simulink model "torqueControlBalancing"  (Simulink 9.1)
settings: Solver=FixedStepDiscrete  StartTime=0.0  StopTime="Config.SIMULATION_TIME "  FixedStep=Config.tStep  RelTol=1e-3  EnableMultiTasking=on
PostLoadFcn:
  | %% Try to open the static GUI and try to adjust it
  | try
  | 
  |     staticGUI = simulinkStaticGUI;
  | 
  | end
InitFcn:
  | %% initialize the simulation
  | cd(fileparts(which(bdroot)));
  | initTorqueControlBalancing;
  | 
  | %% Try to edit the GUI (the user may have already closed it)
  | try
  | 
  |     %% Update Start Button
  |     set(sl_synch_handles.startButton,'Backgroundcolor',[0.0,1.0,0.0]);
  |     set(sl_synch_handles.startButton,'Enable','on');
  | 
  | end
StartFcn:
  | %% Try to edit the GUI (the user may have already closed it)
  | try
  | 
  |     %% Update Start Button
  |     set(sl_synch_handles.startButton,'Backgroundcolor',[0.8,0.8,0.8]);
  |     set(sl_synch_handles.startButton,'Enable','off');
  | 
  |     %% Update Compile Button
  |     set(sl_synch_handles.compileButton,'Backgroundcolor',[0.8,0.8,0.8]);
  |     set(sl_synch_handles.compileButton,'Enable','off');
  | 
  |     %% Update Exit Button
  |     set(sl_synch_handles.exitButton,'Backgroundcolor',[0.8,0.8,0.8]);
  |     set(sl_synch_handles.exitButton,'Enable','off');
  | 
  | end
StopFcn:
  | %% stop the simulation
  | cd(fileparts(which(bdroot)));
  | stopTorqueControlBalancing;
  | 
  | %% Try to edit the GUI (the user may have already closed it)
  | try
  | 
  |     %% Update Compile Button
  |     set(sl_synch_handles.compileButton,'Backgroundcolor',[1.0,0.6,0.0]);
  |     set(sl_synch_handles.compileButton,'Enable','on');
  | 
  |     %% Update Exit Button
  |     set(sl_synch_handles.exitButton,'Backgroundcolor',[0.0,1.0,1.0]);
  |     set(sl_synch_handles.exitButton,'Enable','on');
  | 
  | end
undefined symbols (not defined in the file or in its folder): bVectorConstraints, Config, ConstraintsMatrix, Gain, Reg, ROBOT_DOF, Sat, StateMachine
libraries: WBToolboxLibrary x77
(part 2 of 2)

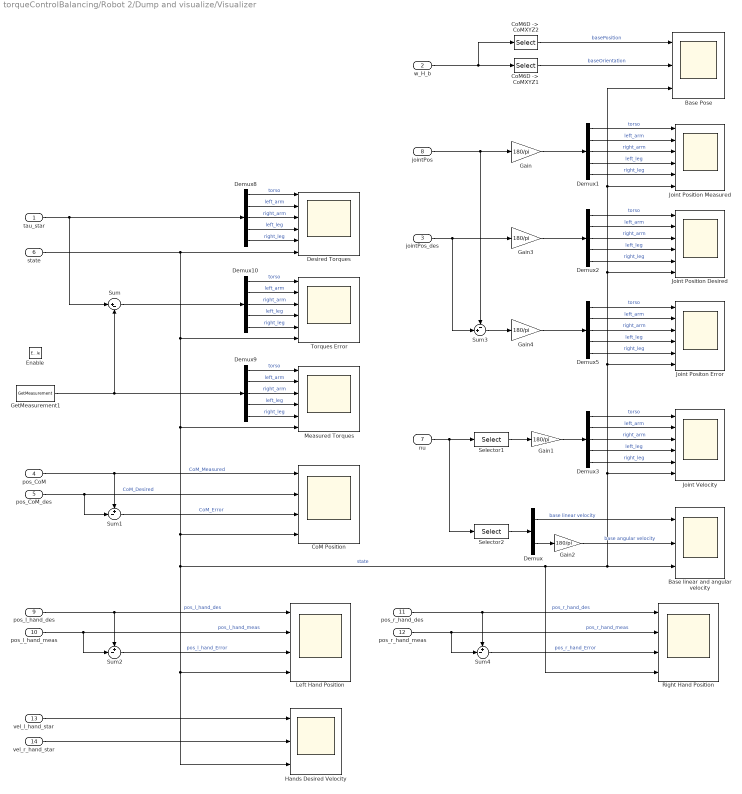
== system torqueControlBalancing/Robot 2/Dump and visualize/Visualizer ==
  tau_star : Inport
  w_H_b : Inport  Port=2
  jointPos_des : Inport  Port=3
  pos_CoM : Inport  Port=4
  pos_CoM_des : Inport  Port=5
  state : Inport  Port=6
  nu : Inport  Port=7
  jointPos : Inport  Port=8
  pos_l_hand_des : Inport  Port=9
  pos_l_hand_meas : Inport  Port=10
  pos_r_hand_des : Inport  Port=11
  pos_r_hand_meas : Inport  Port=12
  vel_l_hand_star : Inport  Port=13
  vel_r_hand_star : Inport  Port=14
  Enable : EnablePort
  Base Pose : Scope  NumInputPorts=3
  Base linear and angular velocity : Scope  NumInputPorts=3
  CoM Position : Scope  NumInputPorts=4
  "CoM6D ->  CoMXYZ1" : Selector  NumberOfDimensions=2  InputPortWidth=7  IndexOptions=Index vector (dialog),Index vector (dialog)  Indices=[1 2 3],[1 2 3]  OutputSizes=1,1
  "CoM6D ->  CoMXYZ2" : Selector  NumberOfDimensions=2  InputPortWidth=7  IndexOptions=Index vector (dialog),Index vector (dialog)  Indices=[1 2 3],[4]  OutputSizes=1,1
  Demux : Demux  Outputs=2
  Demux{1..3,5,8..10} (7 alike) : Demux  Outputs=Config.numOfJointsForEachControlboard
  Desired Torques : Scope  NumInputPorts=6
  Gain{,1..4} (5 alike) : Gain  Gain=180/pi
  GetMeasurement1 : WBToolboxLibrary/States/GetMeasurement  measuredType=Joints Torque
      settings: SourceProductName=WholeBodyToolbox
  Hands Desired Velocity : Scope  NumInputPorts=3
  Joint Position Desired : Scope  NumInputPorts=6
  Joint Position Measured : Scope  NumInputPorts=6
  Joint Positon Error : Scope  NumInputPorts=6
  Joint Velocity : Scope  NumInputPorts=6
  Left Hand Position : Scope  NumInputPorts=4
  Measured Torques : Scope  NumInputPorts=6
  Right Hand Position : Scope  NumInputPorts=4
  Selector1 : Selector  InputPortWidth=6+ROBOT_DOF  IndexOptions=Index vector (dialog)  Indices=[7:6+ROBOT_DOF]  OutputSizes=1
  Selector2 : Selector  InputPortWidth=6+ROBOT_DOF  IndexOptions=Index vector (dialog)  Indices=[1:6]  OutputSizes=1
  Sum : Sum  Inputs=|+-
  Sum1 : Sum  Inputs=+-|
  Sum2 : Sum  Inputs=+-|
  Sum3 : Sum  Inputs=-+|
  Sum4 : Sum  Inputs=+-|
  Torques Error : Scope  NumInputPorts=6
  wires:
  pos_CoM/1 -> Sum1/1, CoM Position/1  "CoM_Measured"
  Gain/1 -> Demux1/1
  jointPos/1 -> Gain/1, Sum3/1
  Demux1/5 -> Joint Position Measured/5  "right_leg"
  Demux1/1 -> Joint Position Measured/1  "torso"
  Demux1/2 -> Joint Position Measured/2  "left_arm"
  Demux1/4 -> Joint Position Measured/4  "left_leg"
  Demux1/3 -> Joint Position Measured/3  "right_arm"
  GetMeasurement1/1 -> Sum/2, Demux9/1
  Demux8/5 -> Desired Torques/5  "right_leg"
  Demux8/1 -> Desired Torques/1  "torso"
  Demux8/2 -> Desired Torques/2  "left_arm"
  Demux8/4 -> Desired Torques/4  "left_leg"
  Demux8/3 -> Desired Torques/3  "right_arm"
  Demux10/5 -> Torques Error/5  "right_leg"
  Demux10/1 -> Torques Error/1  "torso"
  Demux10/2 -> Torques Error/2  "left_arm"
  Demux10/4 -> Torques Error/4  "left_leg"
  Demux10/3 -> Torques Error/3  "right_arm"
  Sum/1 -> Demux10/1
  Demux9/5 -> Measured Torques/5  "right_leg"
  Demux9/1 -> Measured Torques/1  "torso"
  Demux9/2 -> Measured Torques/2  "left_arm"
  Demux9/4 -> Measured Torques/4  "left_leg"
  Demux9/3 -> Measured Torques/3  "right_arm"
  jointPos_des/1 -> Sum3/2, Gain3/1
  Gain3/1 -> Demux2/1
  Demux2/5 -> Joint Position Desired/5  "right_leg"
  Demux2/1 -> Joint Position Desired/1  "torso"
  Demux2/2 -> Joint Position Desired/2  "left_arm"
  Demux2/4 -> Joint Position Desired/4  "left_leg"
  Demux2/3 -> Joint Position Desired/3  "right_arm"
  Gain4/1 -> Demux5/1
  Demux5/5 -> Joint Positon Error/5  "right_leg"
  Demux5/1 -> Joint Positon Error/1  "torso"
  Demux5/2 -> Joint Positon Error/2  "left_arm"
  Demux5/4 -> Joint Positon Error/4  "left_leg"
  Demux5/3 -> Joint Positon Error/3  "right_arm"
  Sum3/1 -> Gain4/1
  pos_CoM_des/1 -> Sum1/2, CoM Position/2  "CoM_Desired"
  w_H_b/1 -> "CoM6D ->  CoMXYZ2"/1, "CoM6D ->  CoMXYZ1"/1
  "CoM6D ->  CoMXYZ2"/1 -> Base Pose/1  "basePosition"
  "CoM6D ->  CoMXYZ1"/1 -> Base Pose/2  "baseOrientation"
  tau_star/1 -> Sum/1, Demux8/1
  nu/1 -> Selector1/1, Selector2/1
  Selector2/1 -> Demux/1
  Gain1/1 -> Demux3/1
  Demux/1 -> Base linear and angular velocity/1  "base linear velocity"
  Gain2/1 -> Base linear and angular velocity/2  "base angular velocity"
  Demux3/3 -> Joint Velocity/3  "right_arm"
  Demux3/5 -> Joint Velocity/5  "right_leg"
  Selector1/1 -> Gain1/1
  Demux3/1 -> Joint Velocity/1  "torso"
  Demux3/2 -> Joint Velocity/2  "left_arm"
  Demux3/4 -> Joint Velocity/4  "left_leg"
  Demux/2 -> Gain2/1
  Sum1/1 -> CoM Position/3  "CoM_Error"
  pos_l_hand_des/1 -> Left Hand Position/1, Sum2/1  "pos_l_hand_des"
  pos_l_hand_meas/1 -> Sum2/2, Left Hand Position/2  "pos_l_hand_meas"
  Sum2/1 -> Left Hand Position/3  "pos_l_hand_Error"
  pos_r_hand_meas/1 -> Sum4/2, Right Hand Position/2  "pos_r_hand_meas"
  pos_r_hand_des/1 -> Right Hand Position/1, Sum4/1  "pos_r_hand_des"
  state/1 -> Left Hand Position/4, Hands Desired Velocity/3, Right Hand Position/4, Base linear and angular velocity/3, Joint Velocity/6, Joint Positon Error/6, Joint Position Desired/6, Base Pose/3, Joint Position Measured/6, CoM Position/4, Measured Torques/6, Torques Error/6, Desired Torques/6  "state"
  Sum4/1 -> Right Hand Position/3  "pos_r_hand_Error"
  vel_l_hand_star/1 -> Hands Desired Velocity/1
  vel_r_hand_star/1 -> Hands Desired Velocity/2

== system torqueControlBalancing/Robot 2/Dynamics and Kinematics/Dynamics ==
  w_H_b : Inport
  jointPos : Inport  Port=2
  nu : Inport  Port=3
  CentroidalMomentum : WBToolboxLibrary/Model/Dynamics/CentroidalMomentum
      settings: SourceProductName=WholeBodyToolbox
  "CoM6D ->  CoMXYZ1" : Selector  InputPortWidth=6+ROBOT_DOF  IndexOptions=Index vector (dialog)  Indices=[7:6+ROBOT_DOF]  OutputSizes=1
  "CoM6D ->  CoMXYZ2" : Selector  InputPortWidth=6+ROBOT_DOF  IndexOptions=Index vector (dialog)  Indices=[1 2 3 4 5 6]  OutputSizes=1
  GetBiasForces : WBToolboxLibrary/Model/Dynamics/GetBiasForces
      settings: SourceProductName=WholeBodyToolbox
  MassMatrix : WBToolboxLibrary/Model/Dynamics/MassMatrix
      settings: SourceProductName=WholeBodyToolbox
  M : Outport
  h : Outport  Port=2
  L : Outport  Port=3
  wires:
  CentroidalMomentum/1 -> L/1
  GetBiasForces/1 -> h/1
  w_H_b/1 -> CentroidalMomentum/1, GetBiasForces/1, MassMatrix/1
  jointPos/1 -> CentroidalMomentum/2, GetBiasForces/2, MassMatrix/2
  "CoM6D ->  CoMXYZ2"/1 -> CentroidalMomentum/3, GetBiasForces/3
  "CoM6D ->  CoMXYZ1"/1 -> CentroidalMomentum/4, GetBiasForces/4
  nu/1 -> "CoM6D ->  CoMXYZ1"/1, "CoM6D ->  CoMXYZ2"/1
  MassMatrix/1 -> M/1

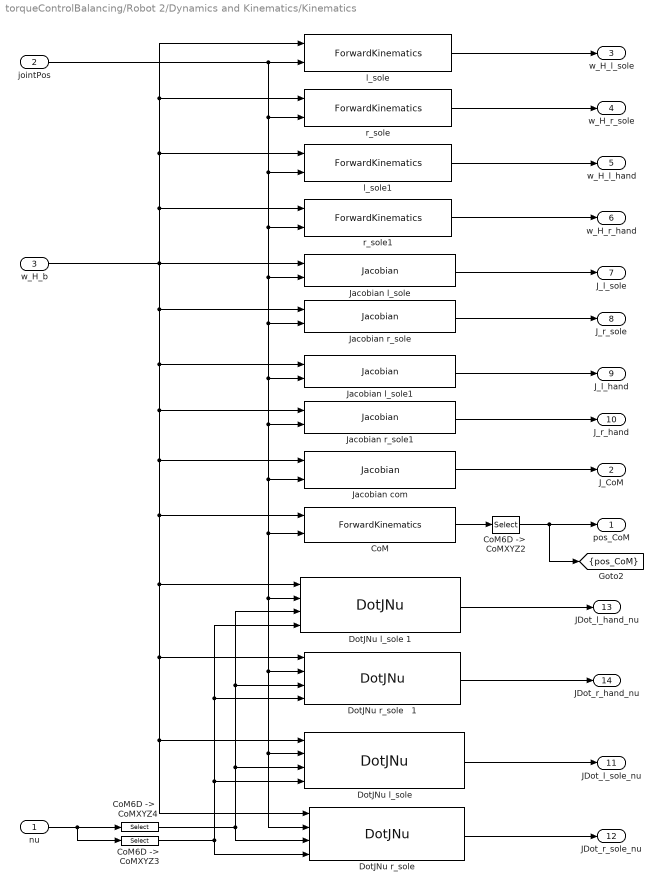
== system torqueControlBalancing/Robot 2/Dynamics and Kinematics/Kinematics ==
  nu : Inport
  jointPos : Inport  Port=2
  w_H_b : Inport  Port=3
  CoM : WBToolboxLibrary/Model/Kinematics/ForwardKinematics  frameName=Frames.COM
      settings: SourceProductName=WholeBodyToolbox
  "CoM6D ->  CoMXYZ2" : Selector  NumberOfDimensions=2  InputPortWidth=7  IndexOptions=Index vector (dialog),Index vector (dialog)  Indices=[1 2 3],[4]  OutputSizes=1,1
  "CoM6D ->  CoMXYZ3" : Selector  InputPortWidth=6+ROBOT_DOF  IndexOptions=Index vector (dialog)  Indices=[7:6+ROBOT_DOF]  OutputSizes=1
  "CoM6D ->  CoMXYZ4" : Selector  InputPortWidth=6+ROBOT_DOF  IndexOptions=Index vector (dialog)  Indices=[1 2 3 4 5 6]  OutputSizes=1
  "DotJNu l_sole " : WBToolboxLibrary/Model/Jacobians/DotJNu  frameName=Frames.LEFT_FOOT
      settings: SourceProductName=WholeBodyToolbox
  DotJNu l_sole 1 : WBToolboxLibrary/Model/Jacobians/DotJNu  frameName=Frames.LEFT_HAND
      settings: SourceProductName=WholeBodyToolbox
  "DotJNu r_sole   " : WBToolboxLibrary/Model/Jacobians/DotJNu  frameName=Frames.RIGHT_FOOT
      settings: SourceProductName=WholeBodyToolbox
  DotJNu r_sole   1 : WBToolboxLibrary/Model/Jacobians/DotJNu  frameName=Frames.RIGHT_HAND
      settings: SourceProductName=WholeBodyToolbox
  Jacobian com : WBToolboxLibrary/Model/Jacobians/Jacobian  frameName=Frames.COM
      settings: SourceProductName=WholeBodyToolbox
  Jacobian l_sole : WBToolboxLibrary/Model/Jacobians/Jacobian  frameName=Frames.LEFT_FOOT
      settings: SourceProductName=WholeBodyToolbox
  Jacobian l_sole1 : WBToolboxLibrary/Model/Jacobians/Jacobian  frameName=Frames.LEFT_HAND
      settings: SourceProductName=WholeBodyToolbox
  Jacobian r_sole : WBToolboxLibrary/Model/Jacobians/Jacobian  frameName=Frames.RIGHT_FOOT
      settings: SourceProductName=WholeBodyToolbox
  Jacobian r_sole1 : WBToolboxLibrary/Model/Jacobians/Jacobian  frameName=Frames.RIGHT_HAND
      settings: SourceProductName=WholeBodyToolbox
  l_sole : WBToolboxLibrary/Model/Kinematics/ForwardKinematics  frameName=Frames.LEFT_FOOT
      settings: SourceProductName=WholeBodyToolbox
  l_sole1 : WBToolboxLibrary/Model/Kinematics/ForwardKinematics  frameName=Frames.LEFT_HAND
      settings: SourceProductName=WholeBodyToolbox
  r_sole : WBToolboxLibrary/Model/Kinematics/ForwardKinematics  frameName=Frames.RIGHT_FOOT
      settings: SourceProductName=WholeBodyToolbox
  r_sole1 : WBToolboxLibrary/Model/Kinematics/ForwardKinematics  frameName=Frames.RIGHT_HAND
      settings: SourceProductName=WholeBodyToolbox
  pos_CoM : Outport
  J_CoM : Outport  Port=2
  w_H_l_sole : Outport  Port=3
  w_H_r_sole : Outport  Port=4
  w_H_l_hand : Outport  Port=5
  w_H_r_hand : Outport  Port=6
  J_l_sole : Outport  Port=7
  J_r_sole : Outport  Port=8
  J_l_hand : Outport  Port=9
  J_r_hand : Outport  Port=10
  JDot_l_sole_nu : Outport  Port=11
  JDot_r_sole_nu : Outport  Port=12
  JDot_l_hand_nu : Outport  Port=13
  JDot_r_hand_nu : Outport  Port=14
  tag scope: pos_CoM=scoped
  wires:
  "CoM6D ->  CoMXYZ3"/1 -> "DotJNu r_sole   "/4, DotJNu l_sole 1/4, DotJNu r_sole   1/4, "DotJNu l_sole "/4
  "CoM6D ->  CoMXYZ4"/1 -> "DotJNu r_sole   "/3, DotJNu r_sole   1/3, DotJNu l_sole 1/3, "DotJNu l_sole "/3
  nu/1 -> "CoM6D ->  CoMXYZ3"/1, "CoM6D ->  CoMXYZ4"/1
  l_sole/1 -> w_H_l_sole/1
  r_sole/1 -> w_H_r_sole/1
  Jacobian l_sole/1 -> J_l_sole/1
  Jacobian r_sole/1 -> J_r_sole/1
  Jacobian com/1 -> J_CoM/1
  CoM/1 -> "CoM6D ->  CoMXYZ2"/1
  "DotJNu l_sole "/1 -> JDot_l_sole_nu/1
  "DotJNu r_sole   "/1 -> JDot_r_sole_nu/1
  "CoM6D ->  CoMXYZ2"/1 -> [pos_CoM], pos_CoM/1
  Jacobian l_sole1/1 -> J_l_hand/1
  Jacobian r_sole1/1 -> J_r_hand/1
  w_H_b/1 -> Jacobian l_sole1/1, Jacobian com/1, DotJNu l_sole 1/1, DotJNu r_sole   1/1, "DotJNu r_sole   "/1, "DotJNu l_sole "/1, CoM/1, Jacobian r_sole1/1, Jacobian r_sole/1, Jacobian l_sole/1, r_sole1/1, l_sole1/1, r_sole/1, l_sole/1
  r_sole1/1 -> w_H_r_hand/1
  l_sole1/1 -> w_H_l_hand/1
  jointPos/1 -> l_sole1/2, r_sole1/2, Jacobian l_sole1/2, Jacobian r_sole1/2, Jacobian com/2, DotJNu l_sole 1/2, DotJNu r_sole   1/2, "DotJNu r_sole   "/2, "DotJNu l_sole "/2, CoM/2, Jacobian r_sole/2, Jacobian l_sole/2, r_sole/2, l_sole/2
  DotJNu r_sole   1/1 -> JDot_r_hand_nu/1
  DotJNu l_sole 1/1 -> JDot_l_hand_nu/1

== system torqueControlBalancing/Robot 2/Robot State and References/Compute State Velocity ==
  jointPos : Inport
  jointVel : Inport  Port=2
  w_H_b : Inport  Port=3
  Compute Base Velocity : MATLAB Function  TreatAsAtomicUnit=on
  Feet Jacobians : Subsystem
  Mux : Mux  Inputs=2
  nu : Outport
  wires:
  jointVel/1 -> Mux/2, Compute Base Velocity/3(jointVel)
  Mux/1 -> nu/1
  Compute Base Velocity/1(nu_b) -> Mux/1
  jointPos/1 -> Feet Jacobians/1(jointPos)
  w_H_b/1 -> Feet Jacobians/2(w_H_b)
  Feet Jacobians/1(J_l_sole) -> Compute Base Velocity/1(J_l_sole)
  Feet Jacobians/2(J_r_sole) -> Compute Base Velocity/2(J_r_sole)

== system torqueControlBalancing/Robot 2/Robot State and References/Compute base to fixed link transform ==
  jointPos : Inport
  Constant7 : Constant  Value=eye(4)
  "LFoot to base link transform " : Subsystem
  Relative transform l_sole_H_base : WBToolboxLibrary/Model/Kinematics/ForwardKinematics  frameName=Frames.LEFT_FOOT
      settings: SourceProductName=WholeBodyToolbox
  fixed_l_sole_H_b : Outport
  tag scope: jointPos=scoped
  wires:
  Constant7/1 -> "LFoot to base link transform "/3(w_H_base_fixed), Relative transform l_sole_H_base/1
  "LFoot to base link transform "/1(link_H_b) -> fixed_l_sole_H_b/1
  Relative transform l_sole_H_base/1 -> "LFoot to base link transform "/2(w_H_link)
  jointPos/1 -> [jointPos], "LFoot to base link transform "/1(jointPos), Relative transform l_sole_H_base/2

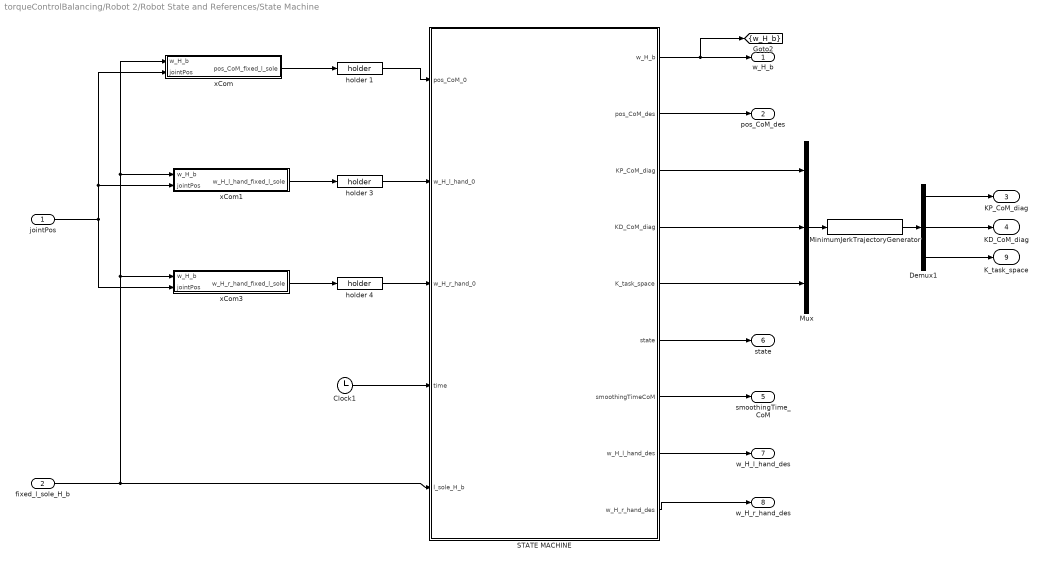
== system torqueControlBalancing/Robot 2/Robot State and References/State Machine ==
  jointPos : Inport
  fixed_l_sole_H_b : Inport  Port=2
  Clock1 : Clock
  Demux1 : Demux  Outputs=[3,3,2]
  MinimumJerkTrajectoryGenerator : WBToolboxLibrary/Utilities/MinimumJerkTrajectoryGenerator  externalSettlingTime=off  settlingTime=Config.SmoothingTimeGainScheduling  sampleTime=Config.tStep  resetOnSettlingTime=off  firstDerivatives=off  secondDerivatives=off  explicitInitialValue=off
      settings: SourceProductName=WholeBodyToolbox
  Mux : Mux  Inputs=3
  STATE MACHINE : MATLAB Function  TreatAsAtomicUnit=on
  holder 1 : WBToolboxLibrary/Utilities/holder 
      settings: SourceProductName=WholeBodyToolbox
  holder 3 : WBToolboxLibrary/Utilities/holder 
      settings: SourceProductName=WholeBodyToolbox
  holder 4 : WBToolboxLibrary/Utilities/holder 
      settings: SourceProductName=WholeBodyToolbox
  xCom : Subsystem
  xCom1 : Subsystem
  xCom3 : Subsystem
  w_H_b : Outport
  pos_CoM_des : Outport  Port=2
  KP_CoM_diag : Outport  Port=3
  KD_CoM_diag : Outport  Port=4
  smoothingTime_CoM : Outport  Port=5
  state : Outport  Port=6
  w_H_l_hand_des : Outport  Port=7
  w_H_r_hand_des : Outport  Port=8
  K_task_space : Outport  Port=9
  tag scope: w_H_b=scoped
  wires:
  xCom/1("pos_CoM_fixed_l_sole ") -> holder 1/1
  STATE MACHINE/2(pos_CoM_des) -> pos_CoM_des/1
  STATE MACHINE/6(state) -> state/1
  STATE MACHINE/3(KP_CoM_diag) -> Mux/1
  STATE MACHINE/4(KD_CoM_diag) -> Mux/2
  Mux/1 -> MinimumJerkTrajectoryGenerator/1
  MinimumJerkTrajectoryGenerator/1 -> Demux1/1
  jointPos/1 -> xCom1/2(jointPos), xCom/2(jointPos), xCom3/2(jointPos)
  fixed_l_sole_H_b/1 -> xCom/1(w_H_b), xCom1/1(w_H_b), xCom3/1(w_H_b), STATE MACHINE/5(l_sole_H_b)
  Clock1/1 -> STATE MACHINE/4(time)
  holder 1/1 -> STATE MACHINE/1(pos_CoM_0)
  STATE MACHINE/7(smoothingTimeCoM) -> smoothingTime_CoM/1
  STATE MACHINE/1(w_H_b) -> [w_H_b], w_H_b/1
  xCom1/1("w_H_l_hand_fixed_l_sole ") -> holder 3/1
  holder 3/1 -> STATE MACHINE/2(w_H_l_hand_0)
  xCom3/1("w_H_r_hand_fixed_l_sole ") -> holder 4/1
  holder 4/1 -> STATE MACHINE/3(w_H_r_hand_0)
  STATE MACHINE/5(K_task_space) -> Mux/3
  STATE MACHINE/8(w_H_l_hand_des) -> w_H_l_hand_des/1
  STATE MACHINE/9(w_H_r_hand_des) -> w_H_r_hand_des/1
  Demux1/1 -> KP_CoM_diag/1
  Demux1/2 -> KD_CoM_diag/1
  Demux1/3 -> K_task_space/1

== system torqueControlBalancing/Robot 2/Robot State and References/Update Gains and References ==
  pos_CoM_des : Inport
  KP_CoM_diag : Inport  Port=2
  KD_CoM_diag : Inport  Port=3
  smoothingTime_CoM : Inport  Port=4
  Reshape Gains Matrices : Subsystem
  Selector1 : Selector  NumberOfDimensions=2  InputPortWidth=3  IndexOptions=Index vector (dialog),Index vector (dialog)  Indices=[1 2 3],[1]  OutputSizes=1,1
  Smooth reference CoM : Subsystem
  KP_CoM : Outport
  KD_CoM : Outport  Port=2
  desired_pos_vel_acc_CoM : Outport  Port=3
  tag scope: pos_CoM_des=scoped
  wires:
  pos_CoM_des/1 -> Smooth reference CoM/1(pos_CoM_des)
  smoothingTime_CoM/1 -> Smooth reference CoM/2(smoothingTime_CoM)
  Smooth reference CoM/1(desired_pos_vel_acc_CoM) -> Selector1/1, desired_pos_vel_acc_CoM/1
  KP_CoM_diag/1 -> Reshape Gains Matrices/1(KP_CoM_diag)
  KD_CoM_diag/1 -> Reshape Gains Matrices/2(KD_CoM_diag)
  Reshape Gains Matrices/1(KP_CoM) -> KP_CoM/1
  Reshape Gains Matrices/2(KD_CoM) -> KD_CoM/1
  Selector1/1 -> [pos_CoM_des]

== system torqueControlBalancing/Robot 2/emergency stop: joint limits/STOP IF JOINTS HIT THE LIMITS ==
  jointPos : Inport
  Enable : EnablePort
  Assertion : Assertion
  GetLimits : WBToolboxLibrary/States/GetLimits  limitsSource=ControlBoard  limitsType=Position
      settings: SourceProductName=WholeBodyToolbox
  MATLAB Function : MATLAB Function  TreatAsAtomicUnit=on
  index1 : Constant  Value=0.01  VectorParams1D=off
  wires:
  jointPos/1 -> MATLAB Function/3(u)
  MATLAB Function/1(inRange) -> Assertion/1
  GetLimits/1 -> MATLAB Function/1(umin)
  GetLimits/2 -> MATLAB Function/2(umax)
  index1/1 -> MATLAB Function/4(tol)

== system torqueControlBalancing/Robot 2/emergency stop: joint limits/STOP IF THERE ARE SPIKES IN THE ENCODERS ==
  jointPos : Inport
  Enable : EnablePort
  Assertion : Assertion
  MATLAB Function : MATLAB Function  TreatAsAtomicUnit=on
  index1 : Constant  Value=Sat.maxJointsPositionDelta  VectorParams1D=off
  wires:
  jointPos/1 -> MATLAB Function/1(u)
  MATLAB Function/1(noSpikes) -> Assertion/1
  index1/1 -> MATLAB Function/2(delta_u_max)

== system torqueControlBalancing/Robot 1/Balancing Controller QP/Compute Desired Torques/QPSolver ==
  HessianMatrixTwoFeet : Inport
  gradientTwoFeet : Inport  Port=2
  ConstraintsMatrixTwoFeet : Inport  Port=3
  bVectorConstraintsTwoFeet : Inport  Port=4
  QP Two Feet : Subsystem  TreatAsAtomicUnit=on
  f_0_twoFeet : Outport
  tag scope: QPStatus=scoped
  wires:
  bVectorConstraintsTwoFeet/1 -> QP Two Feet/4(ubA)
  gradientTwoFeet/1 -> QP Two Feet/2(g)
  ConstraintsMatrixTwoFeet/1 -> QP Two Feet/3(A)
  HessianMatrixTwoFeet/1 -> QP Two Feet/1(H)
  QP Two Feet/1(QPStatus) -> [QPStatus]
  QP Two Feet/2(f0_twoFeet) -> f_0_twoFeet/1

== system torqueControlBalancing/Robot 1/Robot State and References/Compute State Velocity/Feet Jacobians ==
  jointPos : Inport
  w_H_b : Inport  Port=2
  Jacobian l_sole : WBToolboxLibrary/Model/Jacobians/Jacobian  frameName=Frames.LEFT_FOOT
      settings: SourceProductName=WholeBodyToolbox
  Jacobian r_sole : WBToolboxLibrary/Model/Jacobians/Jacobian  frameName=Frames.RIGHT_FOOT
      settings: SourceProductName=WholeBodyToolbox
  J_l_sole : Outport
  J_r_sole : Outport  Port=2
  wires:
  Jacobian l_sole/1 -> J_l_sole/1
  Jacobian r_sole/1 -> J_r_sole/1
  w_H_b/1 -> Jacobian r_sole/1, Jacobian l_sole/1
  jointPos/1 -> Jacobian l_sole/2, Jacobian r_sole/2

== system torqueControlBalancing/Robot 1/Robot State and References/Compute base to fixed link transform/LFoot to base link transform  ==
  jointPos : Inport
  w_H_link : Inport  Port=2
  w_H_base_fixed : Inport  Port=3
  Fixed base to root link transform : WBToolboxLibrary/Model/Kinematics/ForwardKinematics  frameName=Frames.BASE
      settings: SourceProductName=WholeBodyToolbox
  Inv_2 : Product  Inputs=/*  Multiplication=Matrix(*)
  link_H_b : Outport
  wires:
  jointPos/1 -> Fixed base to root link transform/2
  Fixed base to root link transform/1 -> Inv_2/2
  w_H_link/1 -> Inv_2/1
  w_H_base_fixed/1 -> Fixed base to root link transform/1
  Inv_2/1 -> link_H_b/1  "link_H_root"

== system torqueControlBalancing/Robot 1/Robot State and References/State Machine/xCom ==
  w_H_b : Inport
  jointPos : Inport  Port=2
  CoM : WBToolboxLibrary/Model/Kinematics/ForwardKinematics  frameName=Frames.COM
      settings: SourceProductName=WholeBodyToolbox
  "CoM6D ->  CoMXYZ2" : Selector  NumberOfDimensions=2  InputPortWidth=7  IndexOptions=Index vector (dialog),Index vector (dialog)  Indices=[1 2 3],[4]  OutputSizes=1,1
  "pos_CoM_fixed_l_sole " : Outport
  wires:
  jointPos/1 -> CoM/2
  "CoM6D ->  CoMXYZ2"/1 -> "pos_CoM_fixed_l_sole "/1
  CoM/1 -> "CoM6D ->  CoMXYZ2"/1
  w_H_b/1 -> CoM/1

== system torqueControlBalancing/Robot 1/Robot State and References/State Machine/xCom1 ==
  w_H_b : Inport
  jointPos : Inport  Port=2
  Left Hand : WBToolboxLibrary/Model/Kinematics/ForwardKinematics  frameName=Frames.LEFT_HAND
      settings: SourceProductName=WholeBodyToolbox
  "w_H_l_hand_fixed_l_sole " : Outport
  wires:
  jointPos/1 -> Left Hand/2
  Left Hand/1 -> "w_H_l_hand_fixed_l_sole "/1
  w_H_b/1 -> Left Hand/1

== system torqueControlBalancing/Robot 1/Robot State and References/State Machine/xCom3 ==
  w_H_b : Inport
  jointPos : Inport  Port=2
  Right Hand : WBToolboxLibrary/Model/Kinematics/ForwardKinematics  frameName=Frames.RIGHT_HAND
      settings: SourceProductName=WholeBodyToolbox
  "w_H_r_hand_fixed_l_sole " : Outport
  wires:
  jointPos/1 -> Right Hand/2
  Right Hand/1 -> "w_H_r_hand_fixed_l_sole "/1
  w_H_b/1 -> Right Hand/1

== system torqueControlBalancing/Robot 1/Robot State and References/Update Gains and References/Reshape Gains Matrices ==
  KP_CoM_diag : Inport
  KD_CoM_diag : Inport  Port=2
  MATLAB Function1 : MATLAB Function  TreatAsAtomicUnit=on
  MATLAB Function2 : MATLAB Function  TreatAsAtomicUnit=on
  KP_CoM : Outport
  KD_CoM : Outport  Port=2
  wires:
  KP_CoM_diag/1 -> MATLAB Function1/1(d)
  KD_CoM_diag/1 -> MATLAB Function2/1(d)
  MATLAB Function1/1(D) -> KP_CoM/1
  MATLAB Function2/1(D) -> KD_CoM/1

== system torqueControlBalancing/Robot 1/Robot State and References/Update Gains and References/Smooth reference CoM ==
  pos_CoM_des : Inport
  smoothingTime_CoM : Inport  Port=2
  Constant : Constant  Value=zeros(6,1)
  MinimumJerkTrajectoryGenerator2 : WBToolboxLibrary/Utilities/MinimumJerkTrajectoryGenerator  externalSettlingTime=on  settlingTime=0.01  sampleTime=Config.tStep  resetOnSettlingTime=off  firstDerivatives=on  secondDerivatives=on  explicitInitialValue=off
      settings: SourceProductName=WholeBodyToolbox
  Mux : Mux  Inputs=3
  Mux1 : Mux  Inputs=2
  Reshape : Reshape  OutputDimensionality=Customize  OutputDimensions=[3,3]
  SMOOTH_DES_COM : Constant  Value=Config.SMOOTH_COM_DES
  Switch3 : Switch  Criteria=u2 > Threshold
  desired_pos_vel_acc_CoM : Outport
  wires:
  smoothingTime_CoM/1 -> MinimumJerkTrajectoryGenerator2/2
  Switch3/1 -> Reshape/1
  pos_CoM_des/1 -> Mux1/1, MinimumJerkTrajectoryGenerator2/1
  SMOOTH_DES_COM/1 -> Switch3/2
  MinimumJerkTrajectoryGenerator2/3 -> Mux/3
  Mux/1 -> Switch3/1
  MinimumJerkTrajectoryGenerator2/2 -> Mux/2
  Reshape/1 -> desired_pos_vel_acc_CoM/1
  MinimumJerkTrajectoryGenerator2/1 -> Mux/1
  Mux1/1 -> Switch3/3
  Constant/1 -> Mux1/2

== system torqueControlBalancing/Robot 2/Balancing Controller QP/Compute Desired Torques/QPSolver ==
  HessianMatrixTwoFeet : Inport
  gradientTwoFeet : Inport  Port=2
  ConstraintsMatrixTwoFeet : Inport  Port=3
  bVectorConstraintsTwoFeet : Inport  Port=4
  QP Two Feet : Subsystem  TreatAsAtomicUnit=on
  f_0_twoFeet : Outport
  tag scope: QPStatus=scoped
  wires:
  bVectorConstraintsTwoFeet/1 -> QP Two Feet/4(ubA)
  gradientTwoFeet/1 -> QP Two Feet/2(g)
  ConstraintsMatrixTwoFeet/1 -> QP Two Feet/3(A)
  HessianMatrixTwoFeet/1 -> QP Two Feet/1(H)
  QP Two Feet/1(QPStatus) -> [QPStatus]
  QP Two Feet/2(f0_twoFeet) -> f_0_twoFeet/1

== system torqueControlBalancing/Robot 2/Robot State and References/Compute State Velocity/Feet Jacobians ==
  jointPos : Inport
  w_H_b : Inport  Port=2
  Jacobian l_sole : WBToolboxLibrary/Model/Jacobians/Jacobian  frameName=Frames.LEFT_FOOT
      settings: SourceProductName=WholeBodyToolbox
  Jacobian r_sole : WBToolboxLibrary/Model/Jacobians/Jacobian  frameName=Frames.RIGHT_FOOT
      settings: SourceProductName=WholeBodyToolbox
  J_l_sole : Outport
  J_r_sole : Outport  Port=2
  wires:
  Jacobian l_sole/1 -> J_l_sole/1
  Jacobian r_sole/1 -> J_r_sole/1
  w_H_b/1 -> Jacobian r_sole/1, Jacobian l_sole/1
  jointPos/1 -> Jacobian l_sole/2, Jacobian r_sole/2

== system torqueControlBalancing/Robot 2/Robot State and References/Compute base to fixed link transform/LFoot to base link transform  ==
  jointPos : Inport
  w_H_link : Inport  Port=2
  w_H_base_fixed : Inport  Port=3
  Fixed base to root link transform : WBToolboxLibrary/Model/Kinematics/ForwardKinematics  frameName=Frames.BASE
      settings: SourceProductName=WholeBodyToolbox
  Inv_2 : Product  Inputs=/*  Multiplication=Matrix(*)
  link_H_b : Outport
  wires:
  jointPos/1 -> Fixed base to root link transform/2
  Fixed base to root link transform/1 -> Inv_2/2
  w_H_link/1 -> Inv_2/1
  w_H_base_fixed/1 -> Fixed base to root link transform/1
  Inv_2/1 -> link_H_b/1  "link_H_root"

== system torqueControlBalancing/Robot 2/Robot State and References/State Machine/xCom ==
  w_H_b : Inport
  jointPos : Inport  Port=2
  CoM : WBToolboxLibrary/Model/Kinematics/ForwardKinematics  frameName=Frames.COM
      settings: SourceProductName=WholeBodyToolbox
  "CoM6D ->  CoMXYZ2" : Selector  NumberOfDimensions=2  InputPortWidth=7  IndexOptions=Index vector (dialog),Index vector (dialog)  Indices=[1 2 3],[4]  OutputSizes=1,1
  "pos_CoM_fixed_l_sole " : Outport
  wires:
  jointPos/1 -> CoM/2
  "CoM6D ->  CoMXYZ2"/1 -> "pos_CoM_fixed_l_sole "/1
  CoM/1 -> "CoM6D ->  CoMXYZ2"/1
  w_H_b/1 -> CoM/1

== system torqueControlBalancing/Robot 2/Robot State and References/State Machine/xCom1 ==
  w_H_b : Inport
  jointPos : Inport  Port=2
  Left Hand : WBToolboxLibrary/Model/Kinematics/ForwardKinematics  frameName=Frames.LEFT_HAND
      settings: SourceProductName=WholeBodyToolbox
  "w_H_l_hand_fixed_l_sole " : Outport
  wires:
  jointPos/1 -> Left Hand/2
  Left Hand/1 -> "w_H_l_hand_fixed_l_sole "/1
  w_H_b/1 -> Left Hand/1

== system torqueControlBalancing/Robot 2/Robot State and References/State Machine/xCom3 ==
  w_H_b : Inport
  jointPos : Inport  Port=2
  Right Hand : WBToolboxLibrary/Model/Kinematics/ForwardKinematics  frameName=Frames.RIGHT_HAND
      settings: SourceProductName=WholeBodyToolbox
  "w_H_r_hand_fixed_l_sole " : Outport
  wires:
  jointPos/1 -> Right Hand/2
  Right Hand/1 -> "w_H_r_hand_fixed_l_sole "/1
  w_H_b/1 -> Right Hand/1

== system torqueControlBalancing/Robot 2/Robot State and References/Update Gains and References/Reshape Gains Matrices ==
  KP_CoM_diag : Inport
  KD_CoM_diag : Inport  Port=2
  MATLAB Function1 : MATLAB Function  TreatAsAtomicUnit=on
  MATLAB Function2 : MATLAB Function  TreatAsAtomicUnit=on
  KP_CoM : Outport
  KD_CoM : Outport  Port=2
  wires:
  KP_CoM_diag/1 -> MATLAB Function1/1(d)
  KD_CoM_diag/1 -> MATLAB Function2/1(d)
  MATLAB Function1/1(D) -> KP_CoM/1
  MATLAB Function2/1(D) -> KD_CoM/1

== system torqueControlBalancing/Robot 2/Robot State and References/Update Gains and References/Smooth reference CoM ==
  pos_CoM_des : Inport
  smoothingTime_CoM : Inport  Port=2
  Constant : Constant  Value=zeros(6,1)
  MinimumJerkTrajectoryGenerator2 : WBToolboxLibrary/Utilities/MinimumJerkTrajectoryGenerator  externalSettlingTime=on  settlingTime=0.01  sampleTime=Config.tStep  resetOnSettlingTime=off  firstDerivatives=on  secondDerivatives=on  explicitInitialValue=off
      settings: SourceProductName=WholeBodyToolbox
  Mux : Mux  Inputs=3
  Mux1 : Mux  Inputs=2
  Reshape : Reshape  OutputDimensionality=Customize  OutputDimensions=[3,3]
  SMOOTH_DES_COM : Constant  Value=Config.SMOOTH_COM_DES
  Switch3 : Switch  Criteria=u2 > Threshold
  desired_pos_vel_acc_CoM : Outport
  wires:
  smoothingTime_CoM/1 -> MinimumJerkTrajectoryGenerator2/2
  Switch3/1 -> Reshape/1
  pos_CoM_des/1 -> Mux1/1, MinimumJerkTrajectoryGenerator2/1
  SMOOTH_DES_COM/1 -> Switch3/2
  MinimumJerkTrajectoryGenerator2/3 -> Mux/3
  Mux/1 -> Switch3/1
  MinimumJerkTrajectoryGenerator2/2 -> Mux/2
  Reshape/1 -> desired_pos_vel_acc_CoM/1
  MinimumJerkTrajectoryGenerator2/1 -> Mux/1
  Mux1/1 -> Switch3/3
  Constant/1 -> Mux1/2

== system torqueControlBalancing/Robot 1/Balancing Controller QP/Compute Desired Torques/QPSolver/QP Two Feet ==
  H : Inport
  g : Inport  Port=2
  A : Inport  Port=3
  ubA : Inport  Port=4
  Analytical Solution Two Feet (unconstrained) : MATLAB Function  TreatAsAtomicUnit=on
  MatchSignalSizes : WBToolboxLibrary/Utilities/MatchSignalSizes
      settings: SourceProductName=WholeBodyToolbox
  Process QP output : MATLAB Function  TreatAsAtomicUnit=on
  QP Two Feet : WBToolboxLibrary/Utilities/QP  lbA=off  ubA=on  lb=off  ub=off  computeObjVal=off  stopIfFails=off
      settings: SourceProductName=WholeBodyToolbox
  QPStatus : Outport
  f0_twoFeet : Outport  Port=2
  wires:
  QP Two Feet/2 -> Process QP output/3(QPStatus), QPStatus/1
  A/1 -> QP Two Feet/3
  Analytical Solution Two Feet (unconstrained)/1(analyticalSolution) -> Process QP output/1(analyticalSolution)
  Process QP output/1(f_star) -> f0_twoFeet/1
  MatchSignalSizes/1 -> Process QP output/2(primalSolution)
  QP Two Feet/1 -> MatchSignalSizes/2
  H/1 -> QP Two Feet/1, Analytical Solution Two Feet (unconstrained)/1(H)
  g/1 -> Analytical Solution Two Feet (unconstrained)/2(g), MatchSignalSizes/1, QP Two Feet/2
  ubA/1 -> QP Two Feet/4

== system torqueControlBalancing/Robot 2/Balancing Controller QP/Compute Desired Torques/QPSolver/QP Two Feet ==
  H : Inport
  g : Inport  Port=2
  A : Inport  Port=3
  ubA : Inport  Port=4
  Analytical Solution Two Feet (unconstrained) : MATLAB Function  TreatAsAtomicUnit=on
  MatchSignalSizes : WBToolboxLibrary/Utilities/MatchSignalSizes
      settings: SourceProductName=WholeBodyToolbox
  Process QP output : MATLAB Function  TreatAsAtomicUnit=on
  QP Two Feet : WBToolboxLibrary/Utilities/QP  lbA=off  ubA=on  lb=off  ub=off  computeObjVal=off  stopIfFails=off
      settings: SourceProductName=WholeBodyToolbox
  QPStatus : Outport
  f0_twoFeet : Outport  Port=2
  wires:
  QP Two Feet/2 -> Process QP output/3(QPStatus), QPStatus/1
  A/1 -> QP Two Feet/3
  Analytical Solution Two Feet (unconstrained)/1(analyticalSolution) -> Process QP output/1(analyticalSolution)
  Process QP output/1(f_star) -> f0_twoFeet/1
  MatchSignalSizes/1 -> Process QP output/2(primalSolution)
  QP Two Feet/1 -> MatchSignalSizes/2
  H/1 -> QP Two Feet/1, Analytical Solution Two Feet (unconstrained)/1(H)
  g/1 -> Analytical Solution Two Feet (unconstrained)/2(g), MatchSignalSizes/1, QP Two Feet/2
  ubA/1 -> QP Two Feet/4

== matlab function Robot 1/Robot State and References/Update Gains and References/Reshape Gains Matrices/MATLAB Function1 ==
  data: d input double; D output double
function D = diagonalMatrixFromVectorFCN(d)

    D = wbc.diagonalMatrixFromVector(d);
end

== matlab function Robot 2/Balancing Controller QP/Compute Desired Torques/QPSolver/QP Two Feet/Analytical Solution Two Feet (unconstrained) ==
  data: H input double; analyticalSolution output double; g input double
function analyticalSolution = analyticalSolutionQP_FCN(H,g)

    analyticalSolution = wbc.analyticalSolutionQP(H,g);
end

== matlab function Robot 2/Balancing Controller QP/Compute Desired Torques/QPSolver/QP Two Feet/Process QP output ==
  data: analyticalSolution input double; primalSolution input double; QPStatus input double; f_star output double; Config parameter double
function f_star = processOutputQP_twoFeetFCN(analyticalSolution,primalSolution,QPStatus,Config)

     f_star = processOutputQP_twoFeet(analyticalSolution,primalSolution,QPStatus,Config);
end

== matlab function Robot 1/Robot State and References/Update Gains and References/Reshape Gains Matrices/MATLAB Function2 ==
  data: d input double; D output double
function D = diagonalMatrixFromVectorFCN(d)

    D = wbc.diagonalMatrixFromVector(d);
end

== matlab function Robot 2/Balancing Controller QP/Momentum Based Balancing Controller  ==
  data: HessianMatrixTwoFeet output double; gradientTwoFeet output double; ConstraintsMatrixTwoFeet output double; bVectorConstraintsTwoFeet output double; tauModel output double; Sigma output double; Na output double; f_LDot output double; ConstraintsMatrix input double; bVectorConstraints input double; nu input double; M input double; h input double; L input double; w_H input double; J input double; JDot_nu input double; pos_CoM input double; J_CoM input double; KP_CoM input double; KD_CoM input double; K_task_space input double; desired_pos_vel_acc_CoM input double; w_H_l_hand_des input double; w_H_r_hand_des input double; Reg parameter double; Gain parameter double; Config parameter double
function [HessianMatrixTwoFeet, gradientTwoFeet, ConstraintsMatrixTwoFeet, bVectorConstraintsTwoFeet, ...
          tauModel, Sigma, Na, f_LDot] =  ...
              momentumBasedControllerFCN(ConstraintsMatrix, bVectorConstraints, nu, M, h, L, w_H, J, JDot_nu, ...
                                         pos_CoM, J_CoM, KP_CoM, KD_CoM, K_task_space, desired_pos_vel_acc_CoM, w_H_l_hand_des, w_H_r_hand_des, Reg, Gain, Config )
                                                 
    [HessianMatrixTwoFeet, gradientTwoFeet, ConstraintsMatrixTwoFeet, bVectorConstraintsTwoFeet, ...
     tauModel, Sigma, Na, f_LDot] =  ...
        momentumBasedController(ConstraintsMatrix, bVectorConstraints, nu, M, h, L, w_H, J, JDot_nu, ...
                                         pos_CoM, J_CoM, KP_CoM, KD_CoM, K_task_space, desired_pos_vel_acc_CoM, w_H_l_hand_des, w_H_r_hand_des, Reg, Gain, Config );
end

== matlab function Robot 2/Robot State and References/Compute State Velocity/Compute Base Velocity ==
  data: J_l_sole input double; J_r_sole input double; nu_b output double; jointVel input double; Reg parameter double
function nu_b = computeBaseVelocityFCN(J_l_sole, J_r_sole, jointVel, Reg)

    pinvDamp_baseVel = Reg.pinvDamp_baseVel;
    
    nu_b = wbc.computeBaseVelocityWithFeetContact(J_l_sole, J_r_sole, [1, 1], jointVel, pinvDamp_baseVel);
end

== matlab function Robot 1/Robot State and References/Compute State Velocity/Compute Base Velocity ==
  data: J_l_sole input double; J_r_sole input double; nu_b output double; jointVel input double; Reg parameter double
function nu_b = computeBaseVelocityFCN(J_l_sole, J_r_sole, jointVel, Reg)

    pinvDamp_baseVel = Reg.pinvDamp_baseVel;
    
    nu_b = wbc.computeBaseVelocityWithFeetContact(J_l_sole, J_r_sole, [1, 1], jointVel, pinvDamp_baseVel);
end

== matlab function Robot 2/Robot State and References/State Machine/STATE MACHINE ==
  data: pos_CoM_0 input double; w_H_l_hand_0 input double; w_H_r_hand_0 input double; time input double; w_H_b output double; pos_CoM_des output double; l_sole_H_b input double; StateMachine parameter double; KP_CoM_diag output double; KD_CoM_diag output double; K_task_space output double; Gain parameter double; state output double; smoothingTimeCoM output double; Config parameter double; w_H_l_hand_des output double; w_H_r_hand_des output double
function [w_H_b, pos_CoM_des, KP_CoM_diag, KD_CoM_diag, K_task_space, state, smoothingTimeCoM, w_H_l_hand_des, w_H_r_hand_des] = ...
              stateMachineMomentumControlFCN(pos_CoM_0, w_H_l_hand_0, w_H_r_hand_0, ...
                                             time, l_sole_H_b, StateMachine, Gain, Config)
 
    [w_H_b, pos_CoM_des, KP_CoM_diag, KD_CoM_diag, state, smoothingTimeCoM, w_H_l_hand_des, w_H_r_hand_des, K_task_space] = ...
        stateMachineMomentumControl(pos_CoM_0, w_H_l_hand_0, w_H_r_hand_0, ...
                                    time, l_sole_H_b, StateMachine, Gain, Config);
end

== matlab function Robot 2/Robot State and References/Update Gains and References/Reshape Gains Matrices/MATLAB Function1 ==
  data: d input double; D output double
function D = diagonalMatrixFromVectorFCN(d)

    D = wbc.diagonalMatrixFromVector(d);
end

== matlab function Robot 2/Robot State and References/Update Gains and References/Reshape Gains Matrices/MATLAB Function2 ==
  data: d input double; D output double
function D = diagonalMatrixFromVectorFCN(d)

    D = wbc.diagonalMatrixFromVector(d);
end

== matlab function Robot 2/emergency stop: joint limits/STOP IF JOINTS HIT THE LIMITS/MATLAB Function ==
  data: umin input double; umax input double; u input double; inRange output double; tol input double
function inRange = checkRangeFCN(umin, umax, u, tol)

     inRange = wbc.checkRange(umin, umax, u, tol);
end

== matlab function Robot 2/emergency stop: joint limits/STOP IF THERE ARE SPIKES IN THE ENCODERS/MATLAB Function ==
  data: u input double; delta_u_max input double; noSpikes output double
function noSpikes = checkSpikes(u, delta_u_max)

     noSpikes = wbc.checkSpikes(u, delta_u_max);
end

== matlab function Robot 1/Robot State and References/State Machine/STATE MACHINE ==
  data: pos_CoM_0 input double; w_H_l_hand_0 input double; w_H_r_hand_0 input double; time input double; w_H_b output double; pos_CoM_des output double; l_sole_H_b input double; StateMachine parameter double; KP_CoM_diag output double; KD_CoM_diag output double; K_task_space output double; Gain parameter double; state output double; smoothingTimeCoM output double; Config parameter double; w_H_l_hand_des output double; w_H_r_hand_des output double
function [w_H_b, pos_CoM_des, KP_CoM_diag, KD_CoM_diag, K_task_space, state, smoothingTimeCoM, w_H_l_hand_des, w_H_r_hand_des] = ...
              stateMachineMomentumControlFCN(pos_CoM_0, w_H_l_hand_0, w_H_r_hand_0, ...
                                             time, l_sole_H_b, StateMachine, Gain, Config)
 
    [w_H_b, pos_CoM_des, KP_CoM_diag, KD_CoM_diag, state, smoothingTimeCoM, w_H_l_hand_des, w_H_r_hand_des, K_task_space] = ...
        stateMachineMomentumControl(pos_CoM_0, w_H_l_hand_0, w_H_r_hand_0, ...
                                    time, l_sole_H_b, StateMachine, Gain, Config);
end

== matlab function Robot 1/emergency stop: joint limits/STOP IF THERE ARE SPIKES IN THE ENCODERS/MATLAB Function ==
  data: u input double; delta_u_max input double; noSpikes output double
function noSpikes = checkSpikes(u, delta_u_max)

     noSpikes = wbc.checkSpikes(u, delta_u_max);
end

== matlab function Robot 1/Balancing Controller QP/Momentum Based Balancing Controller  ==
  data: HessianMatrixTwoFeet output double; gradientTwoFeet output double; ConstraintsMatrixTwoFeet output double; bVectorConstraintsTwoFeet output double; tauModel output double; Sigma output double; Na output double; f_LDot output double; ConstraintsMatrix input double; bVectorConstraints input double; nu input double; M input double; h input double; L input double; w_H input double; J input double; JDot_nu input double; pos_CoM input double; J_CoM input double; KP_CoM input double; KD_CoM input double; K_task_space input double; desired_pos_vel_acc_CoM input double; w_H_l_hand_des input double; w_H_r_hand_des input double; Reg parameter double; Gain parameter double; Config parameter double
function [HessianMatrixTwoFeet, gradientTwoFeet, ConstraintsMatrixTwoFeet, bVectorConstraintsTwoFeet, ...
          tauModel, Sigma, Na, f_LDot] =  ...
              momentumBasedControllerFCN(ConstraintsMatrix, bVectorConstraints, nu, M, h, L, w_H, J, JDot_nu, ...
                                         pos_CoM, J_CoM, KP_CoM, KD_CoM, K_task_space, desired_pos_vel_acc_CoM, w_H_l_hand_des, w_H_r_hand_des, Reg, Gain, Config )
                                                 
    [HessianMatrixTwoFeet, gradientTwoFeet, ConstraintsMatrixTwoFeet, bVectorConstraintsTwoFeet, ...
     tauModel, Sigma, Na, f_LDot] =  ...
        momentumBasedController(ConstraintsMatrix, bVectorConstraints, nu, M, h, L, w_H, J, JDot_nu, ...
                                         pos_CoM, J_CoM, KP_CoM, KD_CoM, K_task_space, desired_pos_vel_acc_CoM, w_H_l_hand_des, w_H_r_hand_des, Reg, Gain, Config );
end

== matlab function Robot 1/emergency stop: joint limits/STOP IF JOINTS HIT THE LIMITS/MATLAB Function ==
  data: umin input double; umax input double; u input double; inRange output double; tol input double
function inRange = checkRangeFCN(umin, umax, u, tol)

     inRange = wbc.checkRange(umin, umax, u, tol);
end

== matlab function Robot 1/Balancing Controller QP/Compute Desired Torques/QPSolver/QP Two Feet/Analytical Solution Two Feet (unconstrained) ==
  data: H input double; analyticalSolution output double; g input double
function analyticalSolution = analyticalSolutionQP_FCN(H,g)

    analyticalSolution = wbc.analyticalSolutionQP(H,g);
end

== matlab function Robot 1/Balancing Controller QP/Compute Desired Torques/QPSolver/QP Two Feet/Process QP output ==
  data: analyticalSolution input double; primalSolution input double; QPStatus input double; f_star output double; Config parameter double
function f_star = processOutputQP_twoFeetFCN(analyticalSolution,primalSolution,QPStatus,Config)

     f_star = processOutputQP_twoFeet(analyticalSolution,primalSolution,QPStatus,Config);
end
